simulink model "SVPWM"  (R2018a)
settings: Solver=ode3  StartTime=0.0  StopTime=2  FixedStep=0.000001  RelTol=1e-3
libraries: powerlib x4, simulink x2
settings Model: Creator=Stephen  LastModifiedBy=Stephen

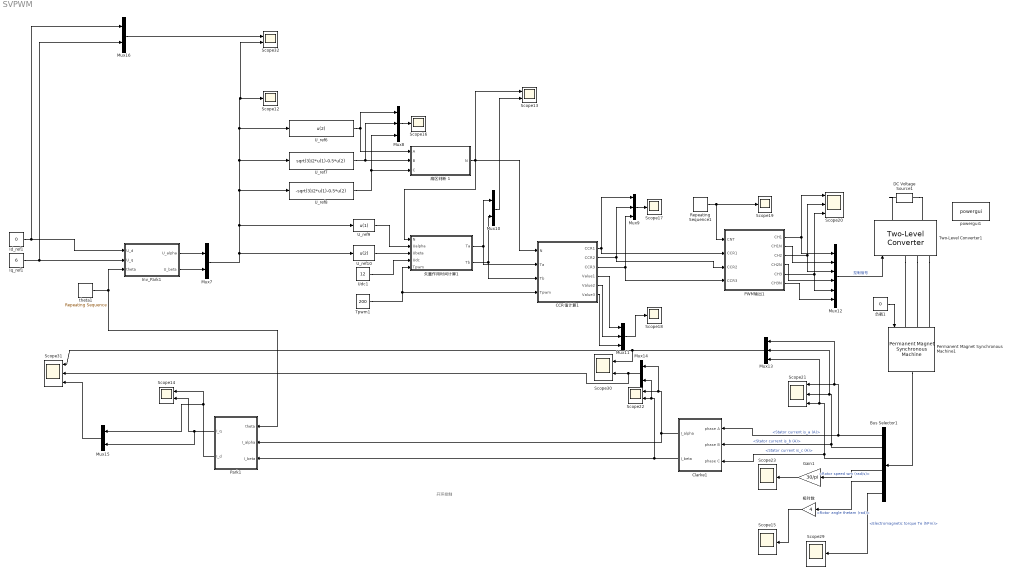
== system SVPWM ==
  note: 开环控制
  Bus Selector1 : BusSelector  OutputSignals=Stator current is_a (A),Stator current is_b (A),Stator current is_c (A),Rotor speed wm (rad/s),Rotor angle thetam (rad),Electromagnetic torque Te (N*m)
  CCR值计算1 : MATLAB Function  TreatAsAtomicUnit=on
  Clarke1 : Subsystem
  DC Voltage Source1 : powerlib/Electrical Sources/DC Voltage Source  Amplitude=12  Measurements=None
  Gain1 : Gain  Gain=30/pi
  Id_ref1 : Constant  Value=0
  Inv_Park1 : Subsystem
  Iq_ref1 : Constant  Value=6
  Mux{7,10,14..16} (5 alike) : Mux  Inputs=2
  Mux{8..9,11,13} (4 alike) : Mux  Inputs=3
  Mux12 : Mux  Inputs=6
  PWM输出1 : MATLAB Function  TreatAsAtomicUnit=on
  Park1 : Subsystem
  Permanent Magnet Synchronous Machine1 : powerlib/Machines/Permanent Magnet Synchronous Machine  NbPhases=3  FluxDistribution=Sinusoidal  RotorType=Round  MechanicalLoad=Torque Tm  PresetModel=No  ShowDetailedParameters=on  MeasurementBus=off  Resistance=0.0485  Inductance=8.5e-3  dqInductances=[8.5e-3,8.5e-3]  La=0.000395  MachineConstant=Flux linkage established by magnets (V.s)  Flux=0.1194  VoltageCst=86.6271  TorqueCst=0.7164  Flat=120  Mechanical=[0.0027 0.0004924 4 0]  PolePairs=4  InitialConditions=[0,0, 0,0]  InitialConditions5ph=[0 0 0 0 0 0]  TsPowergui=0  TsBlock=-1  RefAngle=Aligned with phase A axis (original Park)
      settings: SourceProductName=Simscape Power Systems
  Repeating Sequence1 : simulink/Sources/Repeating Sequence  rep_seq_t=[0 0.00005 0.0001]  rep_seq_y=[0 100 0]
  Scope{12,15..19,23,29} (8 alike) : Scope
  Scope{13..14,22,30,32} (5 alike) : Scope  NumInputPorts=2
  Scope20 : Scope  NumInputPorts=3
  Scope21 : Scope  NumInputPorts=3
  Scope31 : Scope  NumInputPorts=3
  Tpwm1 : Constant  Value=200
  Two-Level Converter1 : powerlib/Power Electronics/Two-Level Converter  ModelType=Switching devices  Ron=1e-3  Rs=1e6  Cs=inf  Vforward=[0,0]  Ron_Diode=1e-3  Rs_Diode=1e6  Cs_Diode=inf  Vf_Diode=1e-3  Rs_CurrentSource=inf
      settings: SourceProductName=Simscape Power Systems  SourceProductBaseCode=PS
  U_ref10 : Fcn  Expr=u(2)
  U_ref6 : Fcn  Expr=u(2)
  U_ref7 : Fcn  Expr=sqrt(3)/2*u(1)-0.5*u(2)
  U_ref8 : Fcn  Expr=-sqrt(3)/2*u(1)-0.5*u(2)
  U_ref9 : Fcn  Expr=u(1)
  Udc1 : Constant  Value=12
  powergui1 : powerlib/powergui  Priority=1  SimulationMode=Continuous  SampleTime=0.000001  frequency=60  Iterations=50  frequencyindice=0  Pbase=100e6  ErrMax=1e-4  UnitsV=kV  UnitsW=MW  buscounter=0  FunctionMessages=off  echomessages=off  EnableUseOfTLC=off  CurrentSourceSwitches=off  DisableSnubberDevices=off  DisableRonSwitches=off  DisableVfSwitches=off  DisplayEquations=off  SolverType=Tustin/Backward Euler (TBE)  Interpol=off  ExternalGateDelay=off  methode=off  Ts=100  x0status=blocks  SPID=on  SwTol=0  HookPort=off  RestoreLinks=warning  ResistiveCurrentMeasurement=off  Frange=[0:2:500]  Ylog=off  Xlog=on  ShowGrid=off  save=off  variable=ZData  structure=0  ZoomFFT=off  StartTime=0.0  cycles=1  DisplayStyle=1  fundamental=60  FreqAxis=off  MaxFrequency=1000  frequencyindicesteady=1  RmsSteady=1  display=off
  theta1 : simulink/Sources/Repeating Sequence  rep_seq_t=[0 0.5]  rep_seq_y=[0 2*pi]
  扇区判断 1 : MATLAB Function  TreatAsAtomicUnit=on
  极对数 : Gain  Gain=4
  矢量作用时间计算1 : MATLAB Function  TreatAsAtomicUnit=on
  负载1 : Constant  Value=0
  wires:
  Permanent Magnet Synchronous Machine1/1 -> Bus Selector1/1
  Park1/1(I_q) -> Mux15/2, Scope14/2
  CCR值计算1/5(Value2) -> Mux11/2
  Bus Selector1/4 -> Gain1/1  "<Rotor speed wm (rad/s)>"
  Park1/2(I_d) -> Mux15/1, Scope14/1
  负载1/1 -> Permanent Magnet Synchronous Machine1/1
  Bus Selector1/1 -> Mux13/1, Scope21/1, Clarke1/1(phase A)  "<Stator current is_a (A)>"
  扇区判断 1/1(N) -> CCR值计算1/1(N), Scope13/1, 矢量作用时间计算1/1(N)
  CCR值计算1/3(CCR3) -> Mux9/3, PWM输出1/4(CCR3)
  PWM输出1/6(CH3N) -> Mux12/6
  Bus Selector1/2 -> Clarke1/2(phase B), Mux13/2, Scope21/2  "<Stator current is_b (A)>"
  Tpwm1/1 -> CCR值计算1/4(Tpwm), 矢量作用时间计算1/5(Tpwm)
  Clarke1/2(I_beta) -> Mux14/2, Scope22/2, Park1/3(I_beta)
  Mux11/1 -> Scope18/1
  Bus Selector1/3 -> Clarke1/3(phase C), Mux13/3, Scope21/3  "<Stator current is_c (A)>"
  Mux12/1 -> Two-Level Converter1/1  "控制信号"
  PWM输出1/5(CH3) -> Mux12/5, Scope20/3
  PWM输出1/3(CH2) -> Mux12/3, Scope20/2
  U_ref7/1 -> Mux8/2, 扇区判断 1/2(B)
  PWM输出1/2(CH1N) -> Mux12/2
  CCR值计算1/2(CCR2) -> PWM输出1/3(CCR2), Mux9/2
  Udc1/1 -> 矢量作用时间计算1/4(Udc)
  矢量作用时间计算1/1(Ta) -> CCR值计算1/2(Ta), Mux10/1
  Repeating Sequence1/1 -> PWM输出1/1(CNT), Scope19/1
  CCR值计算1/4(Value1) -> Mux11/1
  Mux9/1 -> Scope17/1
  Inv_Park1/2(U_beta) -> Mux7/2
  CCR值计算1/6(Value3) -> Mux11/3
  矢量作用时间计算1/2(Tb) -> CCR值计算1/3(Tb), Mux10/2
  Gain1/1 -> Scope23/1
  Clarke1/1(I_alpha) -> Mux14/1, Scope22/1, Park1/2(I_alpha)
  CCR值计算1/1(CCR1) -> PWM输出1/2(CCR1), Mux9/1
  U_ref6/1 -> 扇区判断 1/1(A), Mux8/1
  U_ref8/1 -> Mux8/3, 扇区判断 1/3(C)
  PWM输出1/1(CH1) -> Mux12/1, Scope20/1
  Mux10/1 -> Scope13/2
  Mux8/1 -> Scope16/1
  PWM输出1/4(CH2N) -> Mux12/4
  Inv_Park1/1(U_alpha) -> Mux7/1
  U_ref10/1 -> 矢量作用时间计算1/3(Ubeta)
  U_ref9/1 -> 矢量作用时间计算1/2(Ualpha)
  Iq_ref1/1 -> Mux16/2, Inv_Park1/2(U_q)
  Id_ref1/1 -> Mux16/1, Inv_Park1/1(U_d)
  Bus Selector1/5 -> 极对数/1  "<Rotor angle thetam (rad)>"
  极对数/1 -> Scope15/1
  theta1/1 -> Inv_Park1/3(theta), Park1/1(theta)
  Bus Selector1/6 -> Scope29/1  "<Electromagnetic torque Te (N*m)>"
  Mux14/1 -> Scope31/2, Scope30/2
  Mux13/1 -> Scope31/1, Scope30/1
  Mux15/1 -> Scope31/3
  Mux16/1 -> Scope32/1
  Mux7/1 -> U_ref10/1, U_ref9/1, U_ref7/1, Scope32/2, Scope12/1, U_ref6/1, U_ref8/1
  connections:
  Two-Level Converter1/LConn3 -- Permanent Magnet Synchronous Machine1/LConn3
  Two-Level Converter1/LConn2 -- Permanent Magnet Synchronous Machine1/LConn2
  DC Voltage Source1/RConn1 -- Two-Level Converter1/RConn1
  DC Voltage Source1/LConn1 -- Two-Level Converter1/RConn2
  Two-Level Converter1/LConn1 -- Permanent Magnet Synchronous Machine1/LConn1

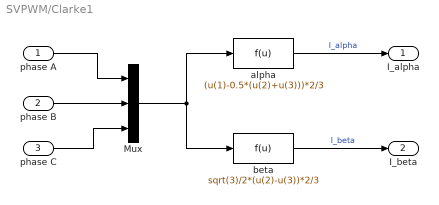
== system SVPWM/Clarke1 ==
  phase A : Inport
  phase B : Inport  Port=2
  phase C : Inport  Port=3
  Mux : Mux  Inputs=3
  alpha : Fcn  Expr=(u(1)-0.5*(u(2)+u(3)))*2/3
  beta : Fcn  Expr=sqrt(3)/2*(u(2)-u(3))*2/3
  I_alpha : Outport
  I_beta : Outport  Port=2
  wires:
  Mux/1 -> alpha/1, beta/1
  alpha/1 -> I_alpha/1  "I_alpha"
  beta/1 -> I_beta/1  "I_beta"
  phase A/1 -> Mux/1
  phase B/1 -> Mux/2
  phase C/1 -> Mux/3

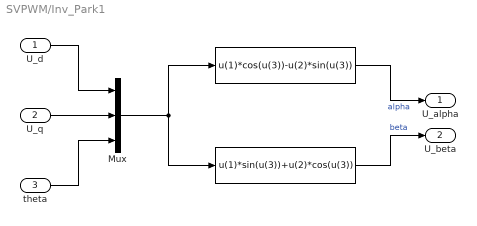
== system SVPWM/Inv_Park1 ==
  U_d : Inport
  U_q : Inport  Port=2
  theta : Inport  Port=3
  " " : Fcn  Expr=u(1)*cos(u(3))-u(2)*sin(u(3))
  "  " : Fcn  Expr=u(1)*sin(u(3))+u(2)*cos(u(3))
  Mux : Mux  Inputs=3
  U_alpha : Outport
  U_beta : Outport  Port=2
  wires:
  "  "/1 -> U_beta/1  "beta"
  Mux/1 -> "  "/1, " "/1
  U_d/1 -> Mux/1
  theta/1 -> Mux/3
  " "/1 -> U_alpha/1  "alpha"
  U_q/1 -> Mux/2

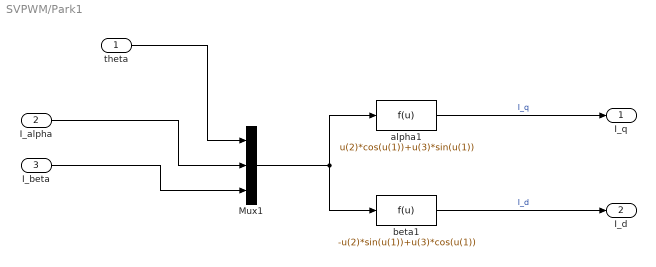
== system SVPWM/Park1 ==
  theta : Inport
  I_alpha : Inport  Port=2
  I_beta : Inport  Port=3
  Mux1 : Mux  Inputs=3
  alpha1 : Fcn  Expr=u(2)*cos(u(1))+u(3)*sin(u(1))
  beta1 : Fcn  Expr=-u(2)*sin(u(1))+u(3)*cos(u(1))
  I_q : Outport
  I_d : Outport  Port=2
  wires:
  I_alpha/1 -> Mux1/2
  Mux1/1 -> beta1/1, alpha1/1
  I_beta/1 -> Mux1/3
  alpha1/1 -> I_q/1  "I_q"
  theta/1 -> Mux1/1
  beta1/1 -> I_d/1  "I_d"

== matlab function SVPWM/CCR值计算1 ==
  data: N input; CCR1 output; Ta input; Tb input; Tpwm input; CCR2 output; CCR3 output; Value1 output; Value2 output; Value3 output
function [CCR1,CCR2,CCR3,Value1,Value2,Value3] = CCRCalculate(N,Ta,Tb,Tpwm)

CCR1=double(0);
CCR2=double(0);
CCR3=double(0);

Value1=(Tpwm-Ta-Tb)/4.0;
Value2=Value1+Ta/2.0;
Value3=Value2+Tb/2.0;

switch(N)
    case 3  %{扇区1 %}
        CCR1=Value1;
        CCR2=Value2;
        CCR3=Value3;

    case 1  %{扇区2%}
        CCR1=Value2;
        CCR2=Value1;
        CCR3=Value3;

    case 5  %{扇区3%}
        CCR1=Value3;
        CCR2=Value1;
        CCR3=Value2;

    case 4  %{扇区4%}
        CCR1=Value3;
        CCR2=Value2;
        CCR3=Value1;

    case 6  %{扇区5%}
        CCR1=Value2;
        CCR2=Value3;
        CCR3=Value1;

    case 2  %{扇区6%}
        CCR1=Value1;
        CCR2=Value3;
        CCR3=Value2;
end

== matlab function SVPWM/PWM输出1 ==
  data: CNT input; CH1 output; CCR1 input; CCR2 input; CCR3 input; CH1N output; CH2 output; CH2N output; CH3 output; CH3N output
function [CH1,CH1N,CH2,CH2N,CH3,CH3N] = PWM(CNT,CCR1,CCR2,CCR3)

if(CNT <= CCR1)
    CH1=0;
    CH1N=1;
else
    CH1=1;
    CH1N=0;
end
if(CNT <= CCR2)
    CH2=0;
    CH2N=1;
else
    CH2=1;
    CH2N=0;
end
if(CNT <= CCR3)
    CH3=0;
    CH3N=1;
else
    CH3=1;
    CH3N=0;
end

== matlab function SVPWM/扇区判断 1 ==
  data: A input; N output; B input; C input
function N = Sector_Judge(A,B,C)
N=0;

if(A>0)
    N=N+1;
end
if(B>0)
    N=N+2;
end
if(C>0)
    N=N+4;
end

== matlab function SVPWM/矢量作用时间计算1 ==
  data: N input; Ta output; Ualpha input; Ubeta input; Udc input; Tpwm input; Tb output
function [Ta,Tb] = VectorCalculate(N,Ualpha,Ubeta,Udc,Tpwm)

Ta=double(0);
Tb=double(0);

X=(sqrt(3)*Tpwm)/Udc*Ubeta;
Y=(sqrt(3)*Tpwm)/Udc*((sqrt(3)/2)*Ualpha+0.5*Ubeta);
Z=(sqrt(3)*Tpwm)/Udc*(-(sqrt(3)/2)*Ualpha+0.5*Ubeta);

if(N==3)  %{扇区1 %}
    Ta=-Z;
    Tb=X;
end
if(N==1)  %{扇区2%}
    Ta=Z;
    Tb=Y;
end
if(N==5)  %{扇区3%}
    Ta=X;
    Tb=-Y;
end
if(N==4)  %{扇区4%}
    Ta=-X;
    Tb=Z;
end
if(N==6)  %{扇区5%}
    Ta=-Y;
    Tb=-Z;
end
if(N==2)  %{扇区6%}
    Ta=Y;
    Tb=-X;
end
Tsum = Ta+Tb;
if(Tsum>Tpwm)  %过调制
    Ta=Tpwm*Ta/Tsum;
    Tb=Tpwm*Tb/Tsum;
end
